simulink subsystem "MyPieroControlVel"  (R2022b)
settings: Solver=VariableStepAuto  StartTime=0.0  StopTime=10.0  RelTol=1e-3
settings Model: Creator=Usuario  LastModifiedBy=Usuario
settings OptimizationCC: ReuseModelBlockBuffer=on
settings RTWCC: GPUComputeCapability=5.0

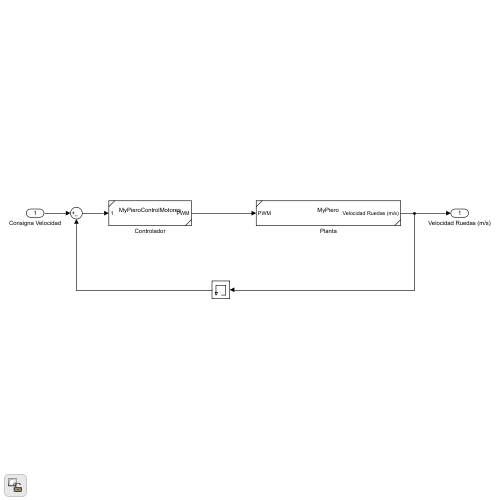
[thumbnail: Simulink's stored preview of the top-level diagram]
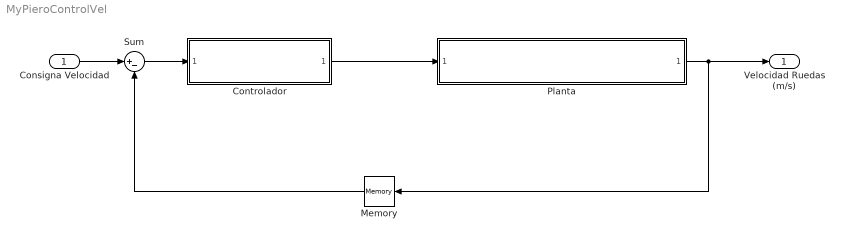
== system MyPieroControlVel ==
  Consigna Velocidad : Inport
  Controlador : Subsystem  ReferencedSubsystem=MyPieroControlMotores
  Memory : Memory
  Planta : Subsystem  ReferencedSubsystem=MyPiero
  Sum : Sum  Inputs=|+-
  Velocidad Ruedas (m/s) : Outport
  wires:
  Planta/1 -> Velocidad Ruedas (m/s)/1, Memory/1
  Memory/1 -> Sum/2
  Sum/1 -> Controlador/1
  Controlador/1 -> Planta/1
  Consigna Velocidad/1 -> Sum/1
